simulink model "simulink_planta"  (R2023a)
settings: Solver=VariableStepAuto  StartTime=0.0  StopTime=80  RelTol=1e-3
undefined symbols (not defined in the file): A, B, C, D
libraries: simulink x1
settings Model: Creator=Agustin  LastModifiedBy=Agustin

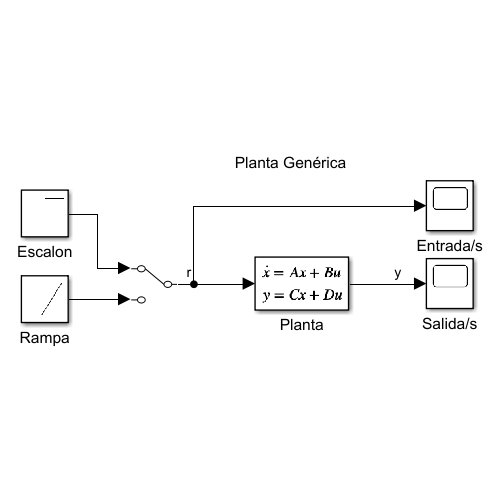
[thumbnail: Simulink's stored preview of the top-level diagram]
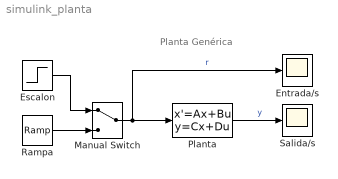
== system simulink_planta ==
  note: Planta Genérica
  Entrada/s : Scope
  Escalon : Step  SampleTime=0
  Manual Switch : ManualSwitch
  Planta : StateSpace  A=A  B=B  C=C  D=D  InitialCondition=0
  Rampa : simulink/Sources/Ramp  slope=1  start=0  InitialOutput=0
  Salida/s : Scope
  wires:
  Planta/1 -> Salida/s/1  "y"
  Escalon/1 -> Manual Switch/1
  Rampa/1 -> Manual Switch/2
  Manual Switch/1 -> Entrada/s/1, Planta/1  "r"
